simulink model "RLFactory"  (R2021a)
settings: Solver=VariableStepAuto  StartTime=0.0  StopTime=1000  RelTol=1e-3
undefined symbols (not defined in the file): BLOCKEDTIMER, GOALSA, GOALSB, GOALSRL, INITAX, INITAY, INITBX, INITBY, MAXVELOA, MAXVELOB, SAFETYDISTANCEA, SAFETYDISTANCEB, THRESHOLDA, THRESHOLDB, TSA, TSB, TSRL
libraries: rllib x1
(part 1 of 2)
settings Model: Creator=julius  LastModifiedBy=juliu
settings SolverCC: AlgebraicLoopSolver=TrustRegion
settings DebuggingCC: SFMachineParentedDataDiag=warning

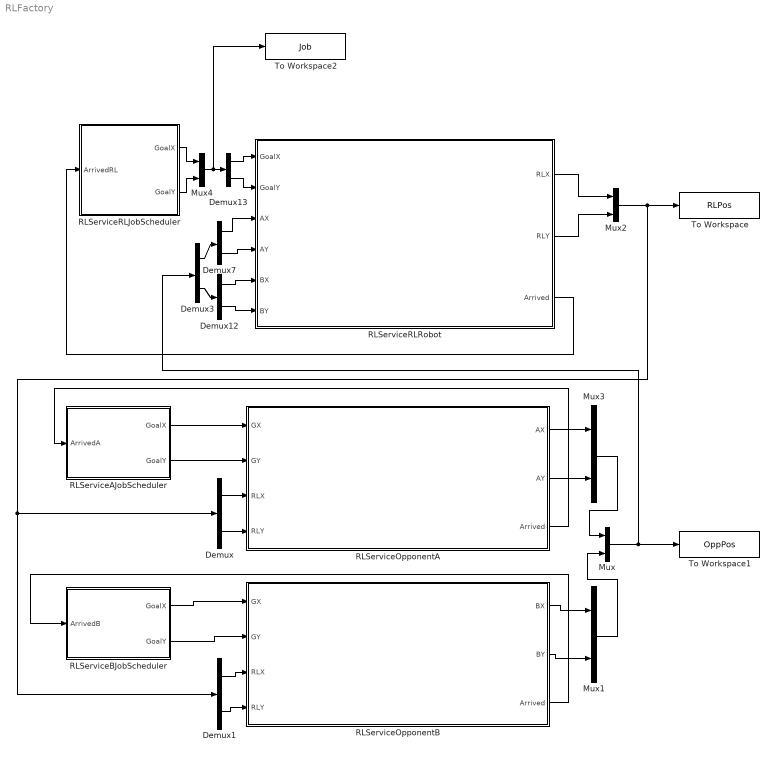
== system RLFactory ==
  Demux{,1,3,7,12..13} (6 alike) : Demux  Outputs=2
  Mux{,1..4} (5 alike) : Mux  Inputs=2
  RLServiceAJobScheduler : Subsystem
  RLServiceBJobScheduler : Subsystem
  RLServiceOpponentA : Subsystem
  RLServiceOpponentB : Subsystem
  RLServiceRLJobScheduler : Subsystem
  RLServiceRLRobot : Subsystem
  To Workspace : ToWorkspace  VariableName=RLPos  SampleTime=TSRL
  To Workspace1 : ToWorkspace  VariableName=OppPos  SampleTime=TSRL
  To Workspace2 : ToWorkspace  VariableName=Job  SampleTime=TSRL
  wires:
  RLServiceAJobScheduler/1(GoalX) -> RLServiceOpponentA/1(GX)
  RLServiceAJobScheduler/2(GoalY) -> RLServiceOpponentA/2(GY)
  RLServiceOpponentA/3(Arrived) -> RLServiceAJobScheduler/1(ArrivedA)
  Demux/1 -> RLServiceOpponentA/3(RLX)
  Demux/2 -> RLServiceOpponentA/4(RLY)
  RLServiceBJobScheduler/1(GoalX) -> RLServiceOpponentB/1(GX)
  RLServiceBJobScheduler/2(GoalY) -> RLServiceOpponentB/2(GY)
  Demux1/1 -> RLServiceOpponentB/3(RLX)
  Demux1/2 -> RLServiceOpponentB/4(RLY)
  RLServiceOpponentB/1(BX) -> Mux1/1
  RLServiceOpponentB/2(BY) -> Mux1/2
  RLServiceOpponentA/1(AX) -> Mux3/1
  RLServiceOpponentA/2(AY) -> Mux3/2
  RLServiceOpponentB/3(Arrived) -> RLServiceBJobScheduler/1(ArrivedB)
  RLServiceRLJobScheduler/2(GoalY) -> Mux4/2
  RLServiceRLJobScheduler/1(GoalX) -> Mux4/1
  Mux3/1 -> Mux/1
  Mux1/1 -> Mux/2
  Demux3/1 -> Demux7/1
  Demux3/2 -> Demux12/1
  Demux13/1 -> RLServiceRLRobot/1(GoalX)
  Demux13/2 -> RLServiceRLRobot/2(GoalY)
  Demux7/1 -> RLServiceRLRobot/3(AX)
  Demux7/2 -> RLServiceRLRobot/4(AY)
  Demux12/1 -> RLServiceRLRobot/5(BX)
  Demux12/2 -> RLServiceRLRobot/6(BY)
  RLServiceRLRobot/3(Arrived) -> RLServiceRLJobScheduler/1(ArrivedRL)
  RLServiceRLRobot/1(RLX) -> Mux2/1
  RLServiceRLRobot/2(RLY) -> Mux2/2
  Mux/1 -> To Workspace1/1, Demux3/1
  Mux2/1 -> To Workspace/1, Demux1/1, Demux/1
  Mux4/1 -> To Workspace2/1, Demux13/1

== system RLFactory/RLServiceAJobScheduler ==
  ArrivedA : Inport
  Constant1 : Constant  Value=GOALSA
  JobScheduler2 : MATLABSystem  System=JobScheduler  SimulateUsing=Interpreted execution
      mask Type: JobScheduler
      mask Display:
      | disp('JobScheduler');
      | port_label('input',1,'workstations');
      | port_label('input',2,'done');
      | port_label('output',1,'currentGoalX');
      | port_label('output',2,'currentGoalY');
  GoalX : Outport
  GoalY : Outport  Port=2
  wires:
  Constant1/1 -> JobScheduler2/1
  JobScheduler2/2 -> GoalY/1
  ArrivedA/1 -> JobScheduler2/2
  JobScheduler2/1 -> GoalX/1

== system RLFactory/RLServiceBJobScheduler ==
  ArrivedB : Inport
  Constant1 : Constant  Value=GOALSB
  JobScheduler2 : MATLABSystem  System=JobScheduler  SimulateUsing=Interpreted execution
      mask Type: JobScheduler
      mask Display:
      | disp('JobScheduler');
      | port_label('input',1,'workstations');
      | port_label('input',2,'done');
      | port_label('output',1,'currentGoalX');
      | port_label('output',2,'currentGoalY');
  GoalX : Outport
  GoalY : Outport  Port=2
  wires:
  Constant1/1 -> JobScheduler2/1
  JobScheduler2/2 -> GoalY/1
  ArrivedB/1 -> JobScheduler2/2
  JobScheduler2/1 -> GoalX/1

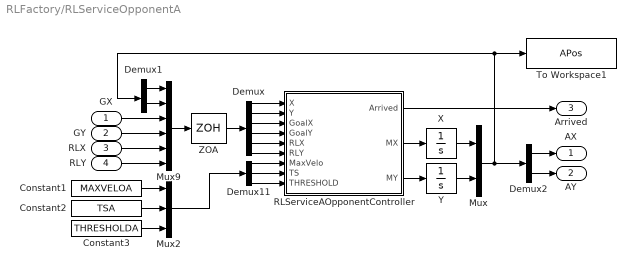
== system RLFactory/RLServiceOpponentA ==
  GX : Inport
  GY : Inport  Port=2
  RLX : Inport  Port=3
  RLY : Inport  Port=4
  Constant1 : Constant  Value=MAXVELOA
  Constant2 : Constant  Value=TSA
  Constant3 : Constant  Value=THRESHOLDA
  Demux : Demux  Outputs=6
  Demux1 : Demux  Outputs=2
  Demux11 : Demux  Outputs=3
  Demux2 : Demux  Outputs=2
  Mux : Mux  Inputs=2
  Mux2 : Mux  Inputs=3
  Mux9 : Mux  Inputs=6
  RLServiceAOpponentController : Subsystem
  To Workspace1 : ToWorkspace  VariableName=APos  SampleTime=0.25
  X : Integrator  InitialCondition=randi(INITAX)
  Y : Integrator  InitialCondition=randi(INITAY)
  ZOA : ZeroOrderHold  SampleTime=TSA
  AX : Outport
  AY : Outport  Port=2
  Arrived : Outport  Port=3
  wires:
  RLServiceAOpponentController/1(Arrived) -> Arrived/1
  Demux/4 -> RLServiceAOpponentController/4(GoalY)
  Demux/6 -> RLServiceAOpponentController/6(RLY)
  X/1 -> Mux/1
  RLY/1 -> Mux9/6
  Demux/5 -> RLServiceAOpponentController/5(RLX)
  GY/1 -> Mux9/4
  Demux/1 -> RLServiceAOpponentController/1(X)
  Y/1 -> Mux/2
  Mux/1 -> Demux1/1, To Workspace1/1, Demux2/1
  Mux9/1 -> ZOA/1
  Demux/3 -> RLServiceAOpponentController/3(GoalX)
  Demux/2 -> RLServiceAOpponentController/2(Y)
  RLX/1 -> Mux9/5
  ZOA/1 -> Demux/1
  GX/1 -> Mux9/3
  Mux2/1 -> Demux11/1
  Demux1/1 -> Mux9/1
  Demux1/2 -> Mux9/2
  Constant2/1 -> Mux2/2
  Constant1/1 -> Mux2/1
  Constant3/1 -> Mux2/3
  Demux2/1 -> AX/1
  Demux2/2 -> AY/1
  RLServiceAOpponentController/3(MY) -> Y/1
  RLServiceAOpponentController/2(MX) -> X/1
  Demux11/1 -> RLServiceAOpponentController/7(MaxVelo)
  Demux11/2 -> RLServiceAOpponentController/8(TS)
  Demux11/3 -> RLServiceAOpponentController/9(THRESHOLD)

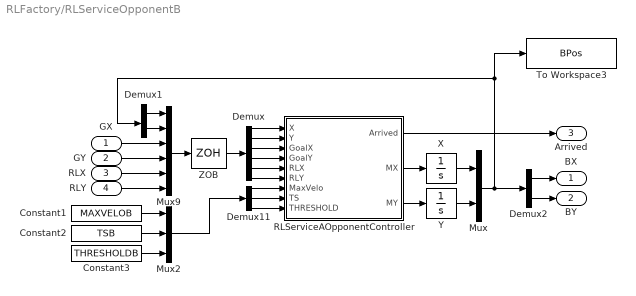
== system RLFactory/RLServiceOpponentB ==
  GX : Inport
  GY : Inport  Port=2
  RLX : Inport  Port=3
  RLY : Inport  Port=4
  Constant1 : Constant  Value=MAXVELOB
  Constant2 : Constant  Value=TSB
  Constant3 : Constant  Value=THRESHOLDB
  Demux : Demux  Outputs=6
  Demux1 : Demux  Outputs=2
  Demux11 : Demux  Outputs=3
  Demux2 : Demux  Outputs=2
  Mux : Mux  Inputs=2
  Mux2 : Mux  Inputs=3
  Mux9 : Mux  Inputs=6
  RLServiceAOpponentController : Subsystem
  To Workspace3 : ToWorkspace  VariableName=BPos  SampleTime=0.25
  X : Integrator  InitialCondition=randi(INITBX)
  Y : Integrator  InitialCondition=randi(INITBY)
  ZOB : ZeroOrderHold  SampleTime=TSB
  BX : Outport
  BY : Outport  Port=2
  Arrived : Outport  Port=3
  wires:
  RLServiceAOpponentController/3(MY) -> Y/1
  RLX/1 -> Mux9/5
  Demux11/1 -> RLServiceAOpponentController/7(MaxVelo)
  Constant2/1 -> Mux2/2
  RLServiceAOpponentController/2(MX) -> X/1
  Mux9/1 -> ZOB/1
  Constant3/1 -> Mux2/3
  Demux1/2 -> Mux9/2
  Demux/1 -> RLServiceAOpponentController/1(X)
  GY/1 -> Mux9/4
  Demux/4 -> RLServiceAOpponentController/4(GoalY)
  RLServiceAOpponentController/1(Arrived) -> Arrived/1
  X/1 -> Mux/1
  Mux/1 -> To Workspace3/1, Demux1/1, Demux2/1
  Demux/6 -> RLServiceAOpponentController/6(RLY)
  Demux/3 -> RLServiceAOpponentController/3(GoalX)
  Demux1/1 -> Mux9/1
  Demux11/2 -> RLServiceAOpponentController/8(TS)
  Demux2/1 -> BX/1
  RLY/1 -> Mux9/6
  Demux/2 -> RLServiceAOpponentController/2(Y)
  Demux11/3 -> RLServiceAOpponentController/9(THRESHOLD)
  ZOB/1 -> Demux/1
  Demux2/2 -> BY/1
  Mux2/1 -> Demux11/1
  Constant1/1 -> Mux2/1
  GX/1 -> Mux9/3
  Y/1 -> Mux/2
  Demux/5 -> RLServiceAOpponentController/5(RLX)

== system RLFactory/RLServiceRLJobScheduler ==
  ArrivedRL : Inport
  Constant : Constant  Value=GOALSRL
  JobScheduler1 : MATLABSystem  System=JobScheduler  SimulateUsing=Code generation
      mask Type: JobScheduler
      mask Display:
      | disp('JobScheduler');
      | port_label('input',1,'workstations');
      | port_label('input',2,'done');
      | port_label('output',1,'currentGoalX');
      | port_label('output',2,'currentGoalY');
  GoalX : Outport
  GoalY : Outport  Port=2
  wires:
  Constant/1 -> JobScheduler1/1
  JobScheduler1/2 -> GoalY/1
  ArrivedRL/1 -> JobScheduler1/2
  JobScheduler1/1 -> GoalX/1

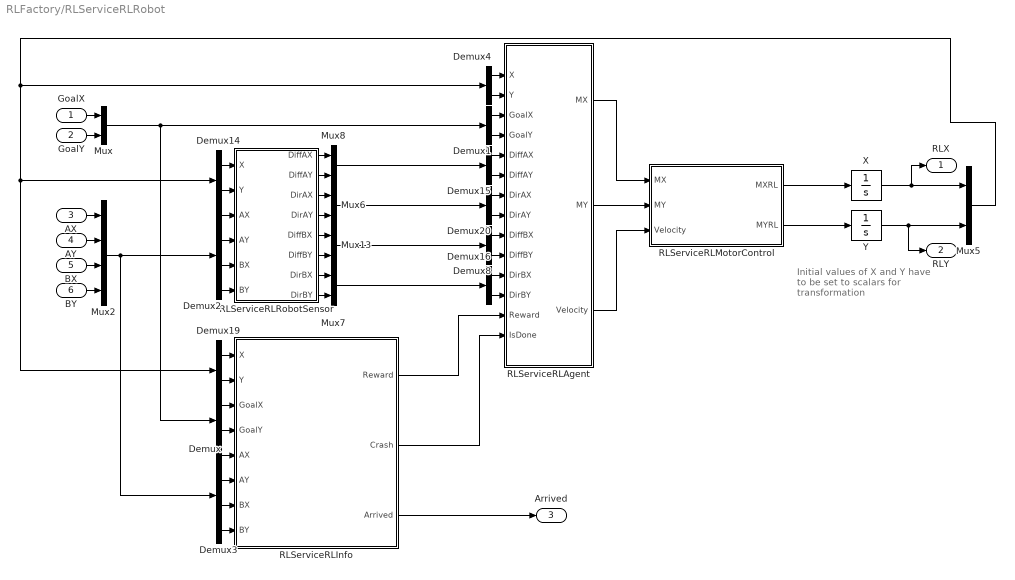
== system RLFactory/RLServiceRLRobot ==
  note: Initial values of X and Y have to be set to scalars for transformation
  GoalX : Inport
  GoalY : Inport  Port=2
  AX : Inport  Port=3
  AY : Inport  Port=4
  BX : Inport  Port=5
  BY : Inport  Port=6
  Demux{,1,4,8,14..16,19..20} (9 alike) : Demux  Outputs=2
  Demux2 : Demux
  Demux3 : Demux
  Mux{,5..8,13} (6 alike) : Mux  Inputs=2
  Mux2 : Mux
  RLServiceRLAgent : Subsystem
  RLServiceRLInfo : Subsystem
  RLServiceRLMotorControl : Subsystem
  RLServiceRLRobotSensor : Subsystem
  X : Integrator  InitialCondition=GOALSRL(1,randi(length(GOALSRL),1))
  Y : Integrator  InitialCondition=GOALSRL(2,randi(length(GOALSRL),1))
  RLX : Outport
  RLY : Outport  Port=2
  Arrived : Outport  Port=3
  wires:
  AX/1 -> Mux2/1
  X/1 -> Mux5/1, RLX/1
  Mux13/1 -> Demux8/1
  Demux2/4 -> RLServiceRLRobotSensor/6(BY)
  Demux4/1 -> RLServiceRLAgent/1(X)
  RLServiceRLRobotSensor/5(DiffBX) -> Mux13/1
  Demux4/2 -> RLServiceRLAgent/2(Y)
  Demux2/1 -> RLServiceRLRobotSensor/3(AX)
  Demux14/2 -> RLServiceRLRobotSensor/2(Y)
  Demux15/1 -> RLServiceRLAgent/5(DiffAX)
  Demux2/2 -> RLServiceRLRobotSensor/4(AY)
  RLServiceRLRobotSensor/4(DirAY) -> Mux6/2
  GoalX/1 -> Mux/1
  Demux20/2 -> RLServiceRLAgent/8(DirAY)
  RLServiceRLRobotSensor/2(DiffAY) -> Mux8/2
  RLServiceRLRobotSensor/7(DirBX) -> Mux7/1
  Mux/1 -> Demux1/1, Demux/1
  Demux2/3 -> RLServiceRLRobotSensor/5(BX)
  Demux1/2 -> RLServiceRLAgent/4(GoalY)
  Demux16/1 -> RLServiceRLAgent/11(DirBX)
  Demux15/2 -> RLServiceRLAgent/6(DiffAY)
  Demux1/1 -> RLServiceRLAgent/3(GoalX)
  Y/1 -> RLY/1, Mux5/2
  RLServiceRLRobotSensor/3(DirAX) -> Mux6/1
  RLServiceRLAgent/2(MY) -> RLServiceRLMotorControl/2(MY)
  Mux2/1 -> Demux3/1, Demux2/1
  Demux20/1 -> RLServiceRLAgent/7(DirAX)
  RLServiceRLRobotSensor/8(DirBY) -> Mux7/2
  Demux8/1 -> RLServiceRLAgent/9(DiffBX)
  BY/1 -> Mux2/4
  GoalY/1 -> Mux/2
  Mux5/1 -> Demux4/1, Demux14/1, Demux19/1
  Mux6/1 -> Demux20/1
  RLServiceRLAgent/1(MX) -> RLServiceRLMotorControl/1(MX)
  RLServiceRLRobotSensor/1(DiffAX) -> Mux8/1
  Mux7/1 -> Demux16/1
  BX/1 -> Mux2/3
  Demux16/2 -> RLServiceRLAgent/12(DirBY)
  AY/1 -> Mux2/2
  Demux8/2 -> RLServiceRLAgent/10(DiffBY)
  Mux8/1 -> Demux15/1
  Demux14/1 -> RLServiceRLRobotSensor/1(X)
  RLServiceRLRobotSensor/6(DiffBY) -> Mux13/2
  RLServiceRLAgent/3(Velocity) -> RLServiceRLMotorControl/3(Velocity)
  RLServiceRLMotorControl/1(MXRL) -> X/1
  RLServiceRLMotorControl/2(MYRL) -> Y/1
  RLServiceRLInfo/2(Crash) -> RLServiceRLAgent/14(IsDone)
  Demux19/1 -> RLServiceRLInfo/1(X)
  Demux19/2 -> RLServiceRLInfo/2(Y)
  Demux/1 -> RLServiceRLInfo/3(GoalX)
  Demux/2 -> RLServiceRLInfo/4(GoalY)
  Demux3/1 -> RLServiceRLInfo/5(AX)
  Demux3/2 -> RLServiceRLInfo/6(AY)
  Demux3/3 -> RLServiceRLInfo/7(BX)
  Demux3/4 -> RLServiceRLInfo/8(BY)
  RLServiceRLInfo/1(Reward) -> RLServiceRLAgent/13(Reward)
  RLServiceRLInfo/3(Arrived) -> Arrived/1

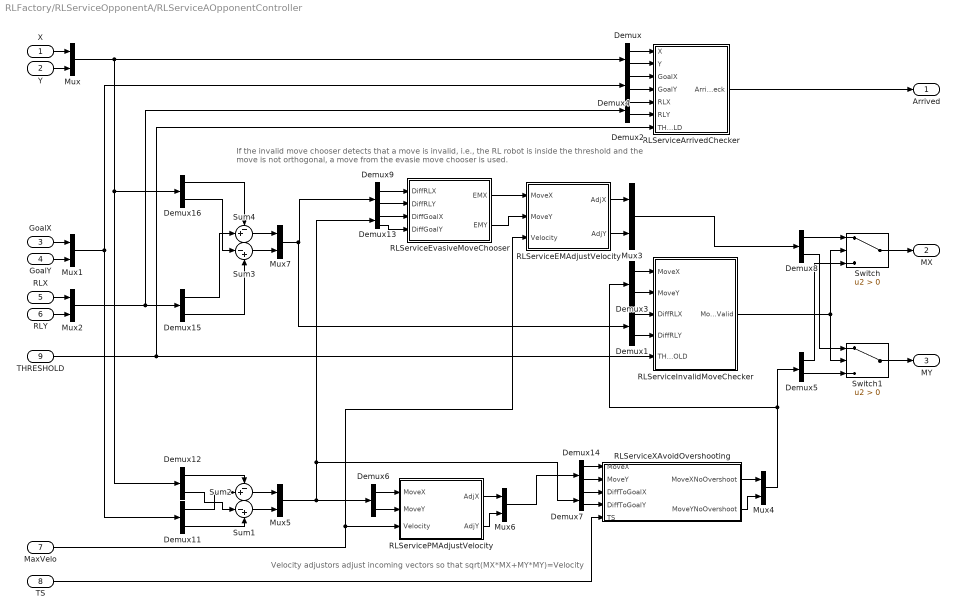
== system RLFactory/RLServiceOpponentA/RLServiceAOpponentController ==
  note: If the invalid move chooser detects that a move is invalid, i.e.,
      | the RL robot is inside the threshold and the move is not orthogonal, a move from the evasie move chooser is used.
  note: Velocity adjustors adjust incoming vectors so that sqrt(MX*MX+MY*MY)=Velocity
  X : Inport
  Y : Inport  Port=2
  GoalX : Inport  Port=3
  GoalY : Inport  Port=4
  RLX : Inport  Port=5
  RLY : Inport  Port=6
  MaxVelo : Inport  Port=7
  TS : Inport  Port=8
  THRESHOLD : Inport  Port=9
  Demux{,1..9,11..16} (16 alike) : Demux  Outputs=2
  Mux{,1..7} (8 alike) : Mux  Inputs=2
  RLServiceArrivedChecker : Subsystem
  RLServiceEMAdjustVelocity : Subsystem
  RLServiceEvasiveMoveChooser : Subsystem
  RLServiceInvalidMoveChecker : Subsystem
  RLServicePMAdjustVelocity : Subsystem
  RLServiceXAvoidOvershooting : Subsystem
  Sum1 : Sum  Inputs=|-+
  Sum2 : Sum  Inputs=-+|
  Sum3 : Sum  Inputs=|-+
  Sum4 : Sum  Inputs=-+|
  Switch : Switch  Criteria=u2 > Threshold
  Switch1 : Switch  Criteria=u2 > Threshold
  Arrived : Outport
  MX : Outport  Port=2
  MY : Outport  Port=3
  wires:
  GoalX/1 -> Mux1/1
  GoalY/1 -> Mux1/2
  RLServiceArrivedChecker/1(ArrivedCheck) -> Arrived/1
  Demux/1 -> RLServiceArrivedChecker/1(X)
  Demux/2 -> RLServiceArrivedChecker/2(Y)
  Demux4/1 -> RLServiceArrivedChecker/3(GoalX)
  Demux4/2 -> RLServiceArrivedChecker/4(GoalY)
  X/1 -> Mux/1
  Y/1 -> Mux/2
  RLX/1 -> Mux2/1
  RLY/1 -> Mux2/2
  Demux3/1 -> RLServiceInvalidMoveChecker/1(MoveX)
  Demux8/1 -> Switch/1
  Demux5/2 -> Switch1/3
  Demux8/2 -> Switch1/1
  THRESHOLD/1 -> RLServiceArrivedChecker/7(THRESHOLD), RLServiceInvalidMoveChecker/5(THRESHOLD)
  Demux3/2 -> RLServiceInvalidMoveChecker/2(MoveY)
  Demux5/1 -> Switch/3
  RLServiceInvalidMoveChecker/1(MoveInValid) -> Switch/2, Switch1/2
  Switch/1 -> MX/1
  Switch1/1 -> MY/1
  Mux5/1 -> Demux6/1, Demux7/1, Demux13/1
  Demux6/2 -> RLServicePMAdjustVelocity/2(MoveY)
  Mux1/1 -> Demux4/1, Demux11/1
  TS/1 -> RLServiceXAvoidOvershooting/5(TS)
  MaxVelo/1 -> RLServiceEMAdjustVelocity/3(Velocity), RLServicePMAdjustVelocity/3(Velocity)
  RLServicePMAdjustVelocity/1(AdjX) -> Mux6/1
  RLServicePMAdjustVelocity/2(AdjY) -> Mux6/2
  RLServiceEvasiveMoveChooser/1(EMX) -> RLServiceEMAdjustVelocity/1(MoveX)
  RLServiceEvasiveMoveChooser/2(EMY) -> RLServiceEMAdjustVelocity/2(MoveY)
  RLServiceEMAdjustVelocity/1(AdjX) -> Mux3/1
  RLServiceEMAdjustVelocity/2(AdjY) -> Mux3/2
  Mux3/1 -> Demux8/1
  RLServiceXAvoidOvershooting/1(MoveXNoOvershoot) -> Mux4/1
  RLServiceXAvoidOvershooting/2(MoveYNoOvershoot) -> Mux4/2
  Mux4/1 -> Demux5/1, Demux3/1
  Sum2/1 -> Mux5/1
  Sum1/1 -> Mux5/2
  Demux6/1 -> RLServicePMAdjustVelocity/1(MoveX)
  Demux7/1 -> RLServiceXAvoidOvershooting/3(DiffToGoalX)
  Demux7/2 -> RLServiceXAvoidOvershooting/4(DiffToGoalY)
  Demux13/1 -> RLServiceEvasiveMoveChooser/3(DiffGoalX)
  Demux13/2 -> RLServiceEvasiveMoveChooser/4(DiffGoalY)
  Demux11/1 -> Sum2/2
  Demux12/2 -> Sum1/1
  Demux11/2 -> Sum1/2
  Demux12/1 -> Sum2/1
  Demux14/1 -> RLServiceXAvoidOvershooting/1(MoveX)
  Demux14/2 -> RLServiceXAvoidOvershooting/2(MoveY)
  Mux6/1 -> Demux14/1
  Sum3/1 -> Mux7/2
  Demux16/1 -> Sum4/1
  Sum4/1 -> Mux7/1
  Mux/1 -> Demux12/1, Demux16/1, Demux/1
  Mux2/1 -> Demux2/1, Demux15/1
  Demux15/2 -> Sum3/2
  Demux15/1 -> Sum4/2
  Demux16/2 -> Sum3/1
  Demux9/1 -> RLServiceEvasiveMoveChooser/1(DiffRLX)
  Demux9/2 -> RLServiceEvasiveMoveChooser/2(DiffRLY)
  Mux7/1 -> Demux1/1, Demux9/1
  Demux1/1 -> RLServiceInvalidMoveChecker/3(DiffRLX)
  Demux1/2 -> RLServiceInvalidMoveChecker/4(DiffRLY)
  Demux2/2 -> RLServiceArrivedChecker/6(RLY)
  Demux2/1 -> RLServiceArrivedChecker/5(RLX)

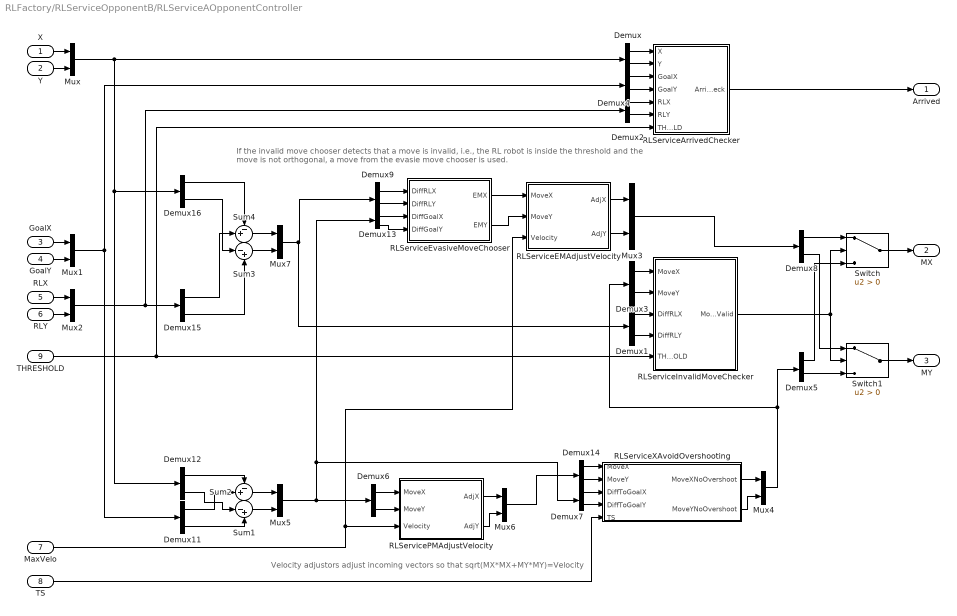
== system RLFactory/RLServiceOpponentB/RLServiceAOpponentController ==
  note: If the invalid move chooser detects that a move is invalid, i.e.,
      | the RL robot is inside the threshold and the move is not orthogonal, a move from the evasie move chooser is used.
  note: Velocity adjustors adjust incoming vectors so that sqrt(MX*MX+MY*MY)=Velocity
  X : Inport
  Y : Inport  Port=2
  GoalX : Inport  Port=3
  GoalY : Inport  Port=4
  RLX : Inport  Port=5
  RLY : Inport  Port=6
  MaxVelo : Inport  Port=7
  TS : Inport  Port=8
  THRESHOLD : Inport  Port=9
  Demux{,1..9,11..16} (16 alike) : Demux  Outputs=2
  Mux{,1..7} (8 alike) : Mux  Inputs=2
  RLServiceArrivedChecker : Subsystem
  RLServiceEMAdjustVelocity : Subsystem
  RLServiceEvasiveMoveChooser : Subsystem
  RLServiceInvalidMoveChecker : Subsystem
  RLServicePMAdjustVelocity : Subsystem
  RLServiceXAvoidOvershooting : Subsystem
  Sum1 : Sum  Inputs=|-+
  Sum2 : Sum  Inputs=-+|
  Sum3 : Sum  Inputs=|-+
  Sum4 : Sum  Inputs=-+|
  Switch : Switch  Criteria=u2 > Threshold
  Switch1 : Switch  Criteria=u2 > Threshold
  Arrived : Outport
  MX : Outport  Port=2
  MY : Outport  Port=3
  wires:
  GoalX/1 -> Mux1/1
  GoalY/1 -> Mux1/2
  RLServiceArrivedChecker/1(ArrivedCheck) -> Arrived/1
  Demux/1 -> RLServiceArrivedChecker/1(X)
  Demux/2 -> RLServiceArrivedChecker/2(Y)
  Demux4/1 -> RLServiceArrivedChecker/3(GoalX)
  Demux4/2 -> RLServiceArrivedChecker/4(GoalY)
  X/1 -> Mux/1
  Y/1 -> Mux/2
  RLX/1 -> Mux2/1
  RLY/1 -> Mux2/2
  Demux3/1 -> RLServiceInvalidMoveChecker/1(MoveX)
  Demux8/1 -> Switch/1
  Demux5/2 -> Switch1/3
  Demux8/2 -> Switch1/1
  THRESHOLD/1 -> RLServiceArrivedChecker/7(THRESHOLD), RLServiceInvalidMoveChecker/5(THRESHOLD)
  Demux3/2 -> RLServiceInvalidMoveChecker/2(MoveY)
  Demux5/1 -> Switch/3
  RLServiceInvalidMoveChecker/1(MoveInValid) -> Switch/2, Switch1/2
  Switch/1 -> MX/1
  Switch1/1 -> MY/1
  Mux5/1 -> Demux6/1, Demux7/1, Demux13/1
  Demux6/2 -> RLServicePMAdjustVelocity/2(MoveY)
  Mux1/1 -> Demux4/1, Demux11/1
  TS/1 -> RLServiceXAvoidOvershooting/5(TS)
  MaxVelo/1 -> RLServiceEMAdjustVelocity/3(Velocity), RLServicePMAdjustVelocity/3(Velocity)
  RLServicePMAdjustVelocity/1(AdjX) -> Mux6/1
  RLServicePMAdjustVelocity/2(AdjY) -> Mux6/2
  RLServiceEvasiveMoveChooser/1(EMX) -> RLServiceEMAdjustVelocity/1(MoveX)
  RLServiceEvasiveMoveChooser/2(EMY) -> RLServiceEMAdjustVelocity/2(MoveY)
  RLServiceEMAdjustVelocity/1(AdjX) -> Mux3/1
  RLServiceEMAdjustVelocity/2(AdjY) -> Mux3/2
  Mux3/1 -> Demux8/1
  RLServiceXAvoidOvershooting/1(MoveXNoOvershoot) -> Mux4/1
  RLServiceXAvoidOvershooting/2(MoveYNoOvershoot) -> Mux4/2
  Mux4/1 -> Demux5/1, Demux3/1
  Sum2/1 -> Mux5/1
  Sum1/1 -> Mux5/2
  Demux6/1 -> RLServicePMAdjustVelocity/1(MoveX)
  Demux7/1 -> RLServiceXAvoidOvershooting/3(DiffToGoalX)
  Demux7/2 -> RLServiceXAvoidOvershooting/4(DiffToGoalY)
  Demux13/1 -> RLServiceEvasiveMoveChooser/3(DiffGoalX)
  Demux13/2 -> RLServiceEvasiveMoveChooser/4(DiffGoalY)
  Demux11/1 -> Sum2/2
  Demux12/2 -> Sum1/1
  Demux11/2 -> Sum1/2
  Demux12/1 -> Sum2/1
  Demux14/1 -> RLServiceXAvoidOvershooting/1(MoveX)
  Demux14/2 -> RLServiceXAvoidOvershooting/2(MoveY)
  Mux6/1 -> Demux14/1
  Sum3/1 -> Mux7/2
  Demux16/1 -> Sum4/1
  Sum4/1 -> Mux7/1
  Mux/1 -> Demux12/1, Demux16/1, Demux/1
  Mux2/1 -> Demux2/1, Demux15/1
  Demux15/2 -> Sum3/2
  Demux15/1 -> Sum4/2
  Demux16/2 -> Sum3/1
  Demux9/1 -> RLServiceEvasiveMoveChooser/1(DiffRLX)
  Demux9/2 -> RLServiceEvasiveMoveChooser/2(DiffRLY)
  Mux7/1 -> Demux1/1, Demux9/1
  Demux1/1 -> RLServiceInvalidMoveChecker/3(DiffRLX)
  Demux1/2 -> RLServiceInvalidMoveChecker/4(DiffRLY)
  Demux2/2 -> RLServiceArrivedChecker/6(RLY)
  Demux2/1 -> RLServiceArrivedChecker/5(RLX)

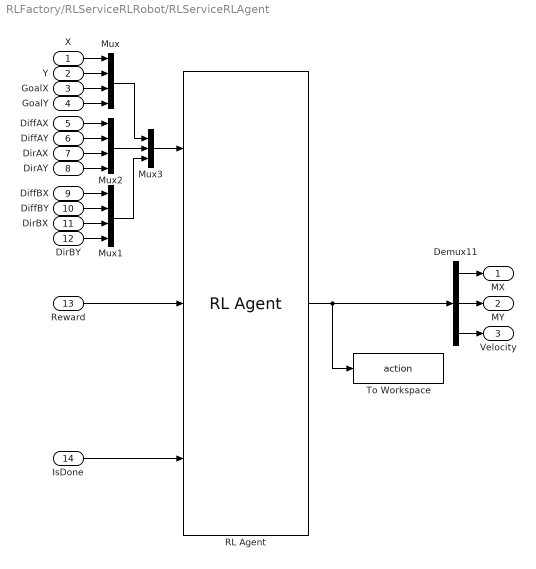
== system RLFactory/RLServiceRLRobot/RLServiceRLAgent ==
  X : Inport
  Y : Inport  Port=2
  GoalX : Inport  Port=3
  GoalY : Inport  Port=4
  DiffAX : Inport  Port=5
  DiffAY : Inport  Port=6
  DirAX : Inport  Port=7
  DirAY : Inport  Port=8
  DiffBX : Inport  Port=9
  DiffBY : Inport  Port=10
  DirBX : Inport  Port=11
  DirBY : Inport  Port=12
  Reward : Inport  Port=13
  IsDone : Inport  Port=14
  Demux11 : Demux  Outputs=3
  Mux : Mux
  Mux1 : Mux
  Mux2 : Mux
  Mux3 : Mux  Inputs=3
  RL Agent : rllib/RL Agent  Agent=qAgent  ProvideReward=on  ProvideIsDone=on  ProvideCumRwd=off  TreatAsDirectFeedthrough=on  CollectLoggedSignals=on  CollectModelStates=on
  To Workspace : ToWorkspace  VariableName=action  SampleTime=-1
  MX : Outport
  MY : Outport  Port=2
  Velocity : Outport  Port=3
  wires:
  IsDone/1 -> RL Agent/3
  Demux11/1 -> MX/1
  Reward/1 -> RL Agent/2
  DirAX/1 -> Mux2/3
  GoalY/1 -> Mux/4
  DiffAX/1 -> Mux2/1
  X/1 -> Mux/1
  GoalX/1 -> Mux/3
  DirAY/1 -> Mux2/4
  DiffAY/1 -> Mux2/2
  Y/1 -> Mux/2
  DiffBX/1 -> Mux1/1
  DiffBY/1 -> Mux1/2
  DirBX/1 -> Mux1/3
  DirBY/1 -> Mux1/4
  Mux2/1 -> Mux3/2
  Mux3/1 -> RL Agent/1
  Mux/1 -> Mux3/1
  Mux1/1 -> Mux3/3
  RL Agent/1 -> To Workspace/1, Demux11/1
  Demux11/2 -> MY/1
  Demux11/3 -> Velocity/1

== system RLFactory/RLServiceRLRobot/RLServiceRLInfo ==
  X : Inport
  Y : Inport  Port=2
  GoalX : Inport  Port=3
  GoalY : Inport  Port=4
  AX : Inport  Port=5
  AY : Inport  Port=6
  BX : Inport  Port=7
  BY : Inport  Port=8
  RLServiceCrashDetector : Subsystem
  RLServiceGoalTracker : Subsystem
  RLServiceReward : Subsystem
  To Workspace1 : ToWorkspace  VariableName=Crash  SampleTime=-1
      settings: MaxDataPoints=1
  Reward : Outport
  Crash : Outport  Port=2
  Arrived : Outport  Port=3
  wires:
  BY/1 -> RLServiceCrashDetector/6(BY)
  GoalY/1 -> RLServiceGoalTracker/4(GoalY)
  AX/1 -> RLServiceCrashDetector/3(AX)
  RLServiceGoalTracker/2(Arrived) -> Arrived/1, RLServiceReward/2(Arrived)
  Y/1 -> RLServiceGoalTracker/2(Y), RLServiceCrashDetector/2(Y)
  GoalX/1 -> RLServiceGoalTracker/3(GoalX)
  BX/1 -> RLServiceCrashDetector/5(BX)
  RLServiceReward/1(Reward) -> Reward/1
  AY/1 -> RLServiceCrashDetector/4(AY)
  X/1 -> RLServiceGoalTracker/1(X), RLServiceCrashDetector/1(X)
  RLServiceGoalTracker/1(Dist) -> RLServiceReward/1(DistGoal)
  RLServiceCrashDetector/2(Crash) -> To Workspace1/1, RLServiceReward/3(Crash), Crash/1
  RLServiceCrashDetector/1(BelowThreshold) -> RLServiceReward/4(BelowThreshold)

== system RLFactory/RLServiceRLRobot/RLServiceRLMotorControl ==
  MX : Inport
  MY : Inport  Port=2
  Velocity : Inport  Port=3
  RLServiceRLAdjustVelocity : Subsystem
  MXRL : Outport
  MYRL : Outport  Port=2
  wires:
  RLServiceRLAdjustVelocity/1(AdjMX) -> MXRL/1
  RLServiceRLAdjustVelocity/2(AdjMY) -> MYRL/1
  MX/1 -> RLServiceRLAdjustVelocity/1(MoveX)
  MY/1 -> RLServiceRLAdjustVelocity/2(MoveY)
  Velocity/1 -> RLServiceRLAdjustVelocity/3(Velocity)

== system RLFactory/RLServiceRLRobot/RLServiceRLRobotSensor ==
  X : Inport
  Y : Inport  Port=2
  AX : Inport  Port=3
  AY : Inport  Port=4
  BX : Inport  Port=5
  BY : Inport  Port=6
  RLServiceARobotSensorSubsystem : Subsystem
  RLServiceBRobotSensorSubsystem : Subsystem
  DiffAX : Outport
  DiffAY : Outport  Port=2
  DirAX : Outport  Port=3
  DirAY : Outport  Port=4
  DiffBX : Outport  Port=5
  DiffBY : Outport  Port=6
  DirBX : Outport  Port=7
  DirBY : Outport  Port=8
  wires:
  RLServiceBRobotSensorSubsystem/3(DirOppX) -> DirBX/1
  BY/1 -> RLServiceBRobotSensorSubsystem/4(OppY)
  BX/1 -> RLServiceBRobotSensorSubsystem/3(OppX)
  RLServiceARobotSensorSubsystem/4(DirOppY) -> DirAY/1
  X/1 -> RLServiceBRobotSensorSubsystem/1(X), RLServiceARobotSensorSubsystem/1(X)
  RLServiceBRobotSensorSubsystem/4(DirOppY) -> DirBY/1
  Y/1 -> RLServiceBRobotSensorSubsystem/2(Y), RLServiceARobotSensorSubsystem/2(Y)
  RLServiceBRobotSensorSubsystem/2(DiffOppY) -> DiffBY/1
  RLServiceARobotSensorSubsystem/3(DirOppX) -> DirAX/1
  RLServiceBRobotSensorSubsystem/1(DiffOppX) -> DiffBX/1
  AX/1 -> RLServiceARobotSensorSubsystem/3(OppX)
  AY/1 -> RLServiceARobotSensorSubsystem/4(OppY)
  RLServiceARobotSensorSubsystem/1(DiffOppX) -> DiffAX/1
  RLServiceARobotSensorSubsystem/2(DiffOppY) -> DiffAY/1

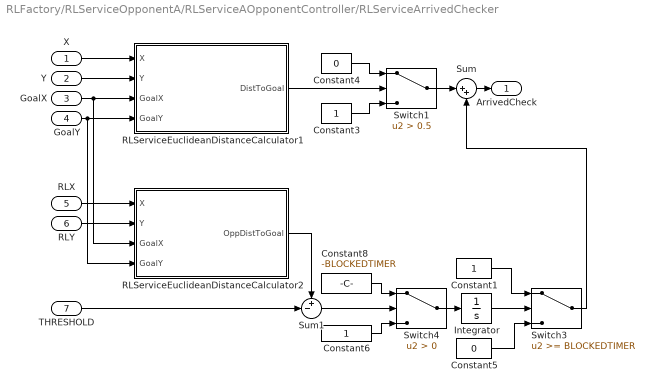
== system RLFactory/RLServiceOpponentA/RLServiceAOpponentController/RLServiceArrivedChecker ==
  X : Inport
  Y : Inport  Port=2
  GoalX : Inport  Port=3
  GoalY : Inport  Port=4
  RLX : Inport  Port=5
  RLY : Inport  Port=6
  THRESHOLD : Inport  Port=7
  Constant1 : Constant
  Constant3 : Constant
  Constant4 : Constant  Value=0
  Constant5 : Constant  Value=0
  Constant6 : Constant
  Constant8 : Constant  Value=-BLOCKEDTIMER
  Integrator : Integrator  LimitOutput=on  UpperSaturationLimit=BLOCKEDTIMER  LowerSaturationLimit=0
  RLServiceEuclideanDistanceCalculator1 : Subsystem
  RLServiceEuclideanDistanceCalculator2 : Subsystem
  Sum : Sum  Inputs=|++
  Sum1 : Sum  Inputs=+-|
  Switch1 : Switch  Criteria=u2 > Threshold  Threshold=0.5
  Switch3 : Switch  Threshold=BLOCKEDTIMER
  Switch4 : Switch  Criteria=u2 > Threshold
  ArrivedCheck : Outport
  wires:
  RLServiceEuclideanDistanceCalculator1/1(DistToGoal) -> Switch1/2
  X/1 -> RLServiceEuclideanDistanceCalculator1/1(X)
  Switch1/1 -> Sum/1
  Constant3/1 -> Switch1/3
  Y/1 -> RLServiceEuclideanDistanceCalculator1/2(Y)
  Constant4/1 -> Switch1/1
  Sum/1 -> ArrivedCheck/1
  Switch3/1 -> Sum/2
  Integrator/1 -> Switch3/2
  Constant5/1 -> Switch3/3
  RLX/1 -> RLServiceEuclideanDistanceCalculator2/1(X)
  RLY/1 -> RLServiceEuclideanDistanceCalculator2/2(Y)
  GoalX/1 -> RLServiceEuclideanDistanceCalculator2/3(GoalX), RLServiceEuclideanDistanceCalculator1/3(GoalX)
  GoalY/1 -> RLServiceEuclideanDistanceCalculator2/4(GoalY), RLServiceEuclideanDistanceCalculator1/4(GoalY)
  RLServiceEuclideanDistanceCalculator2/1(OppDistToGoal) -> Sum1/1
  Constant8/1 -> Switch4/1
  Constant6/1 -> Switch4/3
  THRESHOLD/1 -> Sum1/2
  Sum1/1 -> Switch4/2
  Switch4/1 -> Integrator/1
  Constant1/1 -> Switch3/1

== system RLFactory/RLServiceOpponentA/RLServiceAOpponentController/RLServiceEMAdjustVelocity ==
  MoveX : Inport
  MoveY : Inport  Port=2
  Velocity : Inport  Port=3
  Constant : Constant
  Demux1 : Demux  Outputs=2
  Divide : Product  Inputs=*/
  Divide1 : Product  Inputs=*/
  Mux : Mux  Inputs=2
  Product : Product
  Product3 : Product
  Sqrt1 : Sqrt  SaturateOnIntegerOverflow=on
  Square : Math  Operator=square  SaturateOnIntegerOverflow=on
  Square1 : Math  Operator=square  SaturateOnIntegerOverflow=on
  Sum : Sum  Inputs=+|+
  Switch : Switch  Criteria=u2 > Threshold
  AdjX : Outport
  AdjY : Outport  Port=2
  wires:
  Product/1 -> AdjX/1
  MoveY/1 -> Square1/1, Mux/2
  Mux/1 -> Demux1/1
  Divide1/1 -> Product3/1
  Constant/1 -> Switch/3
  Square1/1 -> Sum/2
  Switch/1 -> Divide1/2, Divide/2
  Velocity/1 -> Product/2, Product3/2
  Sum/1 -> Sqrt1/1
  Square/1 -> Sum/1
  Sqrt1/1 -> Switch/2, Switch/1
  Product3/1 -> AdjY/1
  Demux1/2 -> Divide1/1
  MoveX/1 -> Square/1, Mux/1
  Demux1/1 -> Divide/1
  Divide/1 -> Product/1

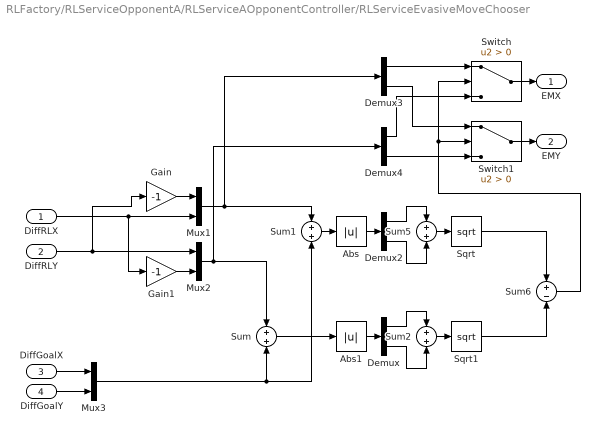
== system RLFactory/RLServiceOpponentA/RLServiceAOpponentController/RLServiceEvasiveMoveChooser ==
  DiffRLX : Inport
  DiffRLY : Inport  Port=2
  DiffGoalX : Inport  Port=3
  DiffGoalY : Inport  Port=4
  Abs : Abs
  Abs1 : Abs
  Demux{,2..4} (4 alike) : Demux  Outputs=2
  Gain : Gain  Gain=-1
  Gain1 : Gain  Gain=-1
  Mux1 : Mux  Inputs=2
  Mux2 : Mux  Inputs=2
  Mux3 : Mux  Inputs=2
  Sqrt : Sqrt  SaturateOnIntegerOverflow=on
  Sqrt1 : Sqrt  SaturateOnIntegerOverflow=on
  Sum{,1..2,5} (4 alike) : Sum  Inputs=+|+
  Sum6 : Sum  Inputs=+|-
  Switch : Switch  Criteria=u2 > Threshold
  Switch1 : Switch  Criteria=u2 > Threshold
  EMX : Outport
  EMY : Outport  Port=2
  wires:
  Gain/1 -> Mux1/1
  DiffRLX/1 -> Gain1/1, Mux1/2
  Gain1/1 -> Mux2/2
  DiffGoalX/1 -> Mux3/1
  DiffGoalY/1 -> Mux3/2
  Mux3/1 -> Sum/2, Sum1/2
  Mux2/1 -> Sum/1, Demux4/1
  Mux1/1 -> Demux3/1, Sum1/1
  Sum1/1 -> Abs/1
  Sum/1 -> Abs1/1
  Abs1/1 -> Demux/1
  Demux/1 -> Sum2/1
  Demux/2 -> Sum2/2
  Demux2/2 -> Sum5/2
  Demux2/1 -> Sum5/1
  Abs/1 -> Demux2/1
  Sum5/1 -> Sqrt/1
  Sum2/1 -> Sqrt1/1
  Sqrt/1 -> Sum6/1
  Sqrt1/1 -> Sum6/2
  Sum6/1 -> Switch/2, Switch1/2
  Demux3/1 -> Switch/1
  Demux3/2 -> Switch1/1
  Demux4/1 -> Switch/3
  Demux4/2 -> Switch1/3
  Switch/1 -> EMX/1
  Switch1/1 -> EMY/1
  DiffRLY/1 -> Mux2/1, Gain/1

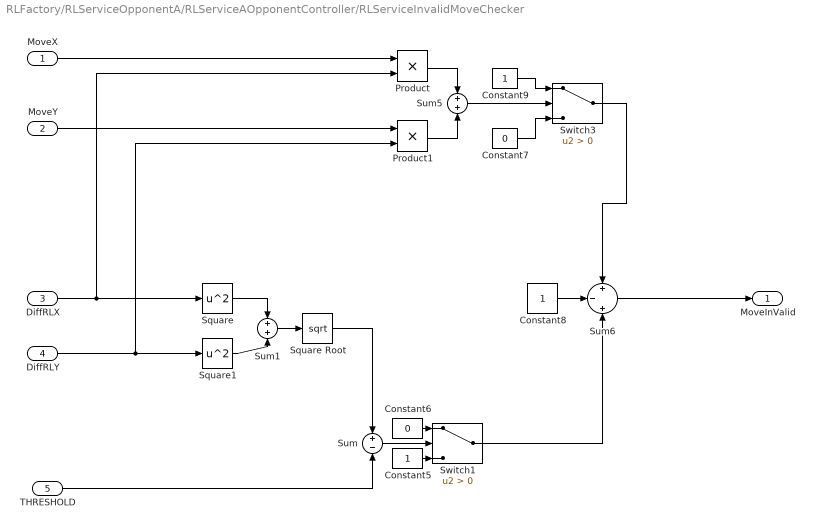
== system RLFactory/RLServiceOpponentA/RLServiceAOpponentController/RLServiceInvalidMoveChecker ==
  MoveX : Inport
  MoveY : Inport  Port=2
  DiffRLX : Inport  Port=3
  DiffRLY : Inport  Port=4
  THRESHOLD : Inport  Port=5
  Constant5 : Constant
  Constant6 : Constant  Value=0
  Constant7 : Constant  Value=0
  Constant8 : Constant
  Constant9 : Constant
  Product : Product
  Product1 : Product
  Square : Math  Operator=square  SaturateOnIntegerOverflow=on
  Square Root : Sqrt  SaturateOnIntegerOverflow=on
  Square1 : Math  Operator=square  SaturateOnIntegerOverflow=on
  Sum : Sum  Inputs=+|-
  Sum1 : Sum
  Sum5 : Sum  Inputs=+|+
  Sum6 : Sum  Inputs=+|-|+
  Switch1 : Switch  Criteria=u2 > Threshold
  Switch3 : Switch  Criteria=u2 > Threshold
  MoveInValid : Outport
  wires:
  Product1/1 -> Sum5/2
  Sum5/1 -> Switch3/2
  Product/1 -> Sum5/1
  Sum6/1 -> MoveInValid/1
  Switch3/1 -> Sum6/1
  Constant9/1 -> Switch3/1
  MoveY/1 -> Product1/1
  MoveX/1 -> Product/1
  Constant8/1 -> Sum6/2
  Constant7/1 -> Switch3/3
  THRESHOLD/1 -> Sum/2
  Sum/1 -> Switch1/2
  Constant5/1 -> Switch1/3
  Constant6/1 -> Switch1/1
  Switch1/1 -> Sum6/3
  DiffRLY/1 -> Square1/1, Product1/2
  DiffRLX/1 -> Product/2, Square/1
  Square1/1 -> Sum1/2
  Sum1/1 -> Square Root/1
  Square/1 -> Sum1/1
  Square Root/1 -> Sum/1

== system RLFactory/RLServiceOpponentA/RLServiceAOpponentController/RLServicePMAdjustVelocity ==
  MoveX : Inport
  MoveY : Inport  Port=2
  Velocity : Inport  Port=3
  Constant : Constant
  Demux1 : Demux  Outputs=2
  Divide : Product  Inputs=*/
  Divide1 : Product  Inputs=*/
  Mux : Mux  Inputs=2
  Product : Product
  Product3 : Product
  Sqrt1 : Sqrt  SaturateOnIntegerOverflow=on
  Square : Math  Operator=square  SaturateOnIntegerOverflow=on
  Square1 : Math  Operator=square  SaturateOnIntegerOverflow=on
  Sum : Sum  Inputs=+|+
  Switch : Switch  Criteria=u2 > Threshold
  AdjX : Outport
  AdjY : Outport  Port=2
  wires:
  Velocity/1 -> Product/2, Product3/2
  MoveX/1 -> Square/1, Mux/1
  MoveY/1 -> Square1/1, Mux/2
  Divide1/1 -> Product3/1
  Divide/1 -> Product/1
  Switch/1 -> Divide1/2, Divide/2
  Constant/1 -> Switch/3
  Mux/1 -> Demux1/1
  Demux1/2 -> Divide1/1
  Square1/1 -> Sum/2
  Sum/1 -> Sqrt1/1
  Demux1/1 -> Divide/1
  Product/1 -> AdjX/1
  Sqrt1/1 -> Switch/2, Switch/1
  Product3/1 -> AdjY/1
  Square/1 -> Sum/1

== system RLFactory/RLServiceOpponentA/RLServiceAOpponentController/RLServiceXAvoidOvershooting ==
  MoveX : Inport
  MoveY : Inport  Port=2
  DiffToGoalX : Inport  Port=3
  DiffToGoalY : Inport  Port=4
  TS : Inport  Port=5
  Abs{1..4} (4 alike) : Abs
  Divide : Product  Inputs=*/
  Divide1 : Product  Inputs=*/
  Product : Product
  Product1 : Product
  Sum1 : Sum  Inputs=-|+
  Sum2 : Sum  Inputs=-|+
  Switch : Switch  Criteria=u2 > Threshold
  Switch1 : Switch  Criteria=u2 > Threshold
  MoveXNoOvershoot : Outport
  MoveYNoOvershoot : Outport  Port=2
  wires:
  Abs1/1 -> Sum1/2
  Switch/1 -> MoveXNoOvershoot/1
  Product/1 -> Abs2/1
  Abs2/1 -> Sum1/1
  DiffToGoalX/1 -> Divide/1, Abs1/1
  Sum1/1 -> Switch/2
  MoveX/1 -> Product/1, Switch/1
  Divide/1 -> Switch/3
  MoveY/1 -> Product1/1, Switch1/1
  Sum2/1 -> Switch1/2
  Abs4/1 -> Sum2/1
  Product1/1 -> Abs4/1
  Divide1/1 -> Switch1/3
  TS/1 -> Divide1/2, Product1/2, Divide/2, Product/2
  Abs3/1 -> Sum2/2
  Switch1/1 -> MoveYNoOvershoot/1
  DiffToGoalY/1 -> Divide1/1, Abs3/1

== system RLFactory/RLServiceOpponentB/RLServiceAOpponentController/RLServiceArrivedChecker ==
  X : Inport
  Y : Inport  Port=2
  GoalX : Inport  Port=3
  GoalY : Inport  Port=4
  RLX : Inport  Port=5
  RLY : Inport  Port=6
  THRESHOLD : Inport  Port=7
  Constant1 : Constant
  Constant3 : Constant
  Constant4 : Constant  Value=0
  Constant5 : Constant  Value=0
  Constant6 : Constant
  Constant8 : Constant  Value=-BLOCKEDTIMER
  Integrator : Integrator  LimitOutput=on  UpperSaturationLimit=BLOCKEDTIMER  LowerSaturationLimit=0
  RLServiceEuclideanDistanceCalculator1 : Subsystem
  RLServiceEuclideanDistanceCalculator2 : Subsystem
  Sum : Sum  Inputs=|++
  Sum1 : Sum  Inputs=+-|
  Switch1 : Switch  Criteria=u2 > Threshold  Threshold=0.5
  Switch3 : Switch  Threshold=BLOCKEDTIMER
  Switch4 : Switch  Criteria=u2 > Threshold
  ArrivedCheck : Outport
  wires:
  RLServiceEuclideanDistanceCalculator1/1(DistToGoal) -> Switch1/2
  X/1 -> RLServiceEuclideanDistanceCalculator1/1(X)
  Switch1/1 -> Sum/1
  Constant3/1 -> Switch1/3
  Y/1 -> RLServiceEuclideanDistanceCalculator1/2(Y)
  Constant4/1 -> Switch1/1
  Sum/1 -> ArrivedCheck/1
  Switch3/1 -> Sum/2
  Integrator/1 -> Switch3/2
  Constant5/1 -> Switch3/3
  RLX/1 -> RLServiceEuclideanDistanceCalculator2/1(X)
  RLY/1 -> RLServiceEuclideanDistanceCalculator2/2(Y)
  GoalX/1 -> RLServiceEuclideanDistanceCalculator2/3(GoalX), RLServiceEuclideanDistanceCalculator1/3(GoalX)
  GoalY/1 -> RLServiceEuclideanDistanceCalculator2/4(GoalY), RLServiceEuclideanDistanceCalculator1/4(GoalY)
  RLServiceEuclideanDistanceCalculator2/1(OppDistToGoal) -> Sum1/1
  Constant8/1 -> Switch4/1
  Constant6/1 -> Switch4/3
  THRESHOLD/1 -> Sum1/2
  Sum1/1 -> Switch4/2
  Switch4/1 -> Integrator/1
  Constant1/1 -> Switch3/1

== system RLFactory/RLServiceOpponentB/RLServiceAOpponentController/RLServiceEMAdjustVelocity ==
  MoveX : Inport
  MoveY : Inport  Port=2
  Velocity : Inport  Port=3
  Constant : Constant
  Demux1 : Demux  Outputs=2
  Divide : Product  Inputs=*/
  Divide1 : Product  Inputs=*/
  Mux : Mux  Inputs=2
  Product : Product
  Product3 : Product
  Sqrt1 : Sqrt  SaturateOnIntegerOverflow=on
  Square : Math  Operator=square  SaturateOnIntegerOverflow=on
  Square1 : Math  Operator=square  SaturateOnIntegerOverflow=on
  Sum : Sum  Inputs=+|+
  Switch : Switch  Criteria=u2 > Threshold
  AdjX : Outport
  AdjY : Outport  Port=2
  wires:
  Product/1 -> AdjX/1
  MoveY/1 -> Square1/1, Mux/2
  Mux/1 -> Demux1/1
  Divide1/1 -> Product3/1
  Constant/1 -> Switch/3
  Square1/1 -> Sum/2
  Switch/1 -> Divide1/2, Divide/2
  Velocity/1 -> Product/2, Product3/2
  Sum/1 -> Sqrt1/1
  Square/1 -> Sum/1
  Sqrt1/1 -> Switch/2, Switch/1
  Product3/1 -> AdjY/1
  Demux1/2 -> Divide1/1
  MoveX/1 -> Square/1, Mux/1
  Demux1/1 -> Divide/1
  Divide/1 -> Product/1

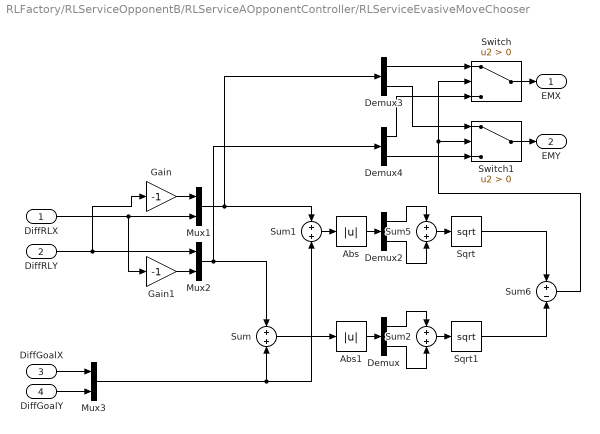
== system RLFactory/RLServiceOpponentB/RLServiceAOpponentController/RLServiceEvasiveMoveChooser ==
  DiffRLX : Inport
  DiffRLY : Inport  Port=2
  DiffGoalX : Inport  Port=3
  DiffGoalY : Inport  Port=4
  Abs : Abs
  Abs1 : Abs
  Demux{,2..4} (4 alike) : Demux  Outputs=2
  Gain : Gain  Gain=-1
  Gain1 : Gain  Gain=-1
  Mux1 : Mux  Inputs=2
  Mux2 : Mux  Inputs=2
  Mux3 : Mux  Inputs=2
  Sqrt : Sqrt  SaturateOnIntegerOverflow=on
  Sqrt1 : Sqrt  SaturateOnIntegerOverflow=on
  Sum{,1..2,5} (4 alike) : Sum  Inputs=+|+
  Sum6 : Sum  Inputs=+|-
  Switch : Switch  Criteria=u2 > Threshold
  Switch1 : Switch  Criteria=u2 > Threshold
  EMX : Outport
  EMY : Outport  Port=2
  wires:
  Gain/1 -> Mux1/1
  DiffRLX/1 -> Gain1/1, Mux1/2
  Gain1/1 -> Mux2/2
  DiffGoalX/1 -> Mux3/1
  DiffGoalY/1 -> Mux3/2
  Mux3/1 -> Sum/2, Sum1/2
  Mux2/1 -> Sum/1, Demux4/1
  Mux1/1 -> Demux3/1, Sum1/1
  Sum1/1 -> Abs/1
  Sum/1 -> Abs1/1
  Abs1/1 -> Demux/1
  Demux/1 -> Sum2/1
  Demux/2 -> Sum2/2
  Demux2/2 -> Sum5/2
  Demux2/1 -> Sum5/1
  Abs/1 -> Demux2/1
  Sum5/1 -> Sqrt/1
  Sum2/1 -> Sqrt1/1
  Sqrt/1 -> Sum6/1
  Sqrt1/1 -> Sum6/2
  Sum6/1 -> Switch/2, Switch1/2
  Demux3/1 -> Switch/1
  Demux3/2 -> Switch1/1
  Demux4/1 -> Switch/3
  Demux4/2 -> Switch1/3
  Switch/1 -> EMX/1
  Switch1/1 -> EMY/1
  DiffRLY/1 -> Mux2/1, Gain/1

== system RLFactory/RLServiceOpponentB/RLServiceAOpponentController/RLServiceInvalidMoveChecker ==
  MoveX : Inport
  MoveY : Inport  Port=2
  DiffRLX : Inport  Port=3
  DiffRLY : Inport  Port=4
  THRESHOLD : Inport  Port=5
  Constant5 : Constant
  Constant6 : Constant  Value=0
  Constant7 : Constant  Value=0
  Constant8 : Constant
  Constant9 : Constant
  Product : Product
  Product1 : Product
  Square : Math  Operator=square  SaturateOnIntegerOverflow=on
  Square Root : Sqrt  SaturateOnIntegerOverflow=on
  Square1 : Math  Operator=square  SaturateOnIntegerOverflow=on
  Sum : Sum  Inputs=+|-
  Sum1 : Sum
  Sum5 : Sum  Inputs=+|+
  Sum6 : Sum  Inputs=+|-|+
  Switch1 : Switch  Criteria=u2 > Threshold
  Switch3 : Switch  Criteria=u2 > Threshold
  MoveInValid : Outport
  wires:
  Product1/1 -> Sum5/2
  Sum5/1 -> Switch3/2
  Product/1 -> Sum5/1
  Sum6/1 -> MoveInValid/1
  Switch3/1 -> Sum6/1
  Constant9/1 -> Switch3/1
  MoveY/1 -> Product1/1
  MoveX/1 -> Product/1
  Constant8/1 -> Sum6/2
  Constant7/1 -> Switch3/3
  THRESHOLD/1 -> Sum/2
  Sum/1 -> Switch1/2
  Constant5/1 -> Switch1/3
  Constant6/1 -> Switch1/1
  Switch1/1 -> Sum6/3
  DiffRLY/1 -> Square1/1, Product1/2
  DiffRLX/1 -> Product/2, Square/1
  Square1/1 -> Sum1/2
  Sum1/1 -> Square Root/1
  Square/1 -> Sum1/1
  Square Root/1 -> Sum/1

== system RLFactory/RLServiceOpponentB/RLServiceAOpponentController/RLServicePMAdjustVelocity ==
  MoveX : Inport
  MoveY : Inport  Port=2
  Velocity : Inport  Port=3
  Constant : Constant
  Demux1 : Demux  Outputs=2
  Divide : Product  Inputs=*/
  Divide1 : Product  Inputs=*/
  Mux : Mux  Inputs=2
  Product : Product
  Product3 : Product
  Sqrt1 : Sqrt  SaturateOnIntegerOverflow=on
  Square : Math  Operator=square  SaturateOnIntegerOverflow=on
  Square1 : Math  Operator=square  SaturateOnIntegerOverflow=on
  Sum : Sum  Inputs=+|+
  Switch : Switch  Criteria=u2 > Threshold
  AdjX : Outport
  AdjY : Outport  Port=2
  wires:
  Velocity/1 -> Product/2, Product3/2
  MoveX/1 -> Square/1, Mux/1
  MoveY/1 -> Square1/1, Mux/2
  Divide1/1 -> Product3/1
  Divide/1 -> Product/1
  Switch/1 -> Divide1/2, Divide/2
  Constant/1 -> Switch/3
  Mux/1 -> Demux1/1
  Demux1/2 -> Divide1/1
  Square1/1 -> Sum/2
  Sum/1 -> Sqrt1/1
  Demux1/1 -> Divide/1
  Product/1 -> AdjX/1
  Sqrt1/1 -> Switch/2, Switch/1
  Product3/1 -> AdjY/1
  Square/1 -> Sum/1

== system RLFactory/RLServiceOpponentB/RLServiceAOpponentController/RLServiceXAvoidOvershooting ==
  MoveX : Inport
  MoveY : Inport  Port=2
  DiffToGoalX : Inport  Port=3
  DiffToGoalY : Inport  Port=4
  TS : Inport  Port=5
  Abs{1..4} (4 alike) : Abs
  Divide : Product  Inputs=*/
  Divide1 : Product  Inputs=*/
  Product : Product
  Product1 : Product
  Sum1 : Sum  Inputs=-|+
  Sum2 : Sum  Inputs=-|+
  Switch : Switch  Criteria=u2 > Threshold
  Switch1 : Switch  Criteria=u2 > Threshold
  MoveXNoOvershoot : Outport
  MoveYNoOvershoot : Outport  Port=2
  wires:
  Abs1/1 -> Sum1/2
  Switch/1 -> MoveXNoOvershoot/1
  Product/1 -> Abs2/1
  Abs2/1 -> Sum1/1
  DiffToGoalX/1 -> Divide/1, Abs1/1
  Sum1/1 -> Switch/2
  MoveX/1 -> Product/1, Switch/1
  Divide/1 -> Switch/3
  MoveY/1 -> Product1/1, Switch1/1
  Sum2/1 -> Switch1/2
  Abs4/1 -> Sum2/1
  Product1/1 -> Abs4/1
  Divide1/1 -> Switch1/3
  TS/1 -> Divide1/2, Product1/2, Divide/2, Product/2
  Abs3/1 -> Sum2/2
  Switch1/1 -> MoveYNoOvershoot/1
  DiffToGoalY/1 -> Divide1/1, Abs3/1

== system RLFactory/RLServiceRLRobot/RLServiceRLInfo/RLServiceCrashDetector ==
  X : Inport
  Y : Inport  Port=2
  AX : Inport  Port=3
  AY : Inport  Port=4
  BX : Inport  Port=5
  BY : Inport  Port=6
  Constant : Constant  Value=SAFETYDISTANCEA
  Constant1 : Constant  Value=SAFETYDISTANCEB
  Constant2 : Constant  Value=THRESHOLDA
  Constant3 : Constant  Value=THRESHOLDB
  Less Than{1..4} (4 alike) : RelationalOperator  Operator=<=  OutDataTypeStr=boolean  RndMeth=Simplest
  Memory : Memory
  OR : Logic  Operator=OR  IconShape=distinctive  AllPortsSameDT=off  OutDataTypeStr=boolean
  OR1 : Logic  Operator=OR  IconShape=distinctive  AllPortsSameDT=off  OutDataTypeStr=boolean
  RLServiceEuclideanDistanceCalculator1 : Subsystem
  RLServiceEuclideanDistanceCalculator2 : Subsystem
  Switch3 : Switch  Criteria=u2 > Threshold
  BelowThreshold : Outport
  Crash : Outport  Port=2
  wires:
  AX/1 -> RLServiceEuclideanDistanceCalculator1/3(XOpp)
  Less Than2/1 -> OR/1
  Memory/1 -> Switch3/1, Switch3/2
  Constant/1 -> Less Than2/2
  Y/1 -> RLServiceEuclideanDistanceCalculator2/2(Y), RLServiceEuclideanDistanceCalculator1/2(Y)
  AY/1 -> RLServiceEuclideanDistanceCalculator1/4(YOpp)
  X/1 -> RLServiceEuclideanDistanceCalculator1/1(X), RLServiceEuclideanDistanceCalculator2/1(X)
  OR/1 -> Switch3/3
  Constant1/1 -> Less Than3/2
  BY/1 -> RLServiceEuclideanDistanceCalculator2/4(YOpp)
  Less Than3/1 -> OR/2
  BX/1 -> RLServiceEuclideanDistanceCalculator2/3(XOpp)
  Constant2/1 -> Less Than1/2
  RLServiceEuclideanDistanceCalculator1/1(Dist) -> Less Than2/1, Less Than1/1
  Constant3/1 -> Less Than4/2
  RLServiceEuclideanDistanceCalculator2/1(Dist) -> Less Than4/1, Less Than3/1
  Less Than1/1 -> OR1/1
  Less Than4/1 -> OR1/2
  Switch3/1 -> Crash/1, Memory/1
  OR1/1 -> BelowThreshold/1

== system RLFactory/RLServiceRLRobot/RLServiceRLInfo/RLServiceGoalTracker ==
  X : Inport
  Y : Inport  Port=2
  GoalX : Inport  Port=3
  GoalY : Inport  Port=4
  Constant1 : Constant
  Constant5 : Constant  Value=0.5
  Constant7 : Constant  Value=0
  Less Than1 : RelationalOperator  Operator=<  OutDataTypeStr=boolean  RndMeth=Simplest
  RLServiceEuclideanDistanceCalculator : Subsystem
  Sum : Sum  Inputs=|++
  Switch : Switch  Criteria=u2 > Threshold
  To Workspace : ToWorkspace  VariableName=Arrived  SampleTime=TSRL
      settings: MaxDataPoints=1
  Unit Delay : UnitDelay  SampleTime=TSRL  HasFrameUpgradeWarning=on
  Zero-Order Hold : ZeroOrderHold  SampleTime=TSRL
  Dist : Outport
  Arrived : Outport  Port=2
  wires:
  Constant7/1 -> Switch/3
  GoalX/1 -> RLServiceEuclideanDistanceCalculator/3(GoalX)
  Y/1 -> RLServiceEuclideanDistanceCalculator/2(Y)
  RLServiceEuclideanDistanceCalculator/1(DistGoal) -> Dist/1, Less Than1/1
  Constant1/1 -> Switch/1
  Switch/1 -> Zero-Order Hold/1
  Less Than1/1 -> Switch/2
  X/1 -> RLServiceEuclideanDistanceCalculator/1(X)
  GoalY/1 -> RLServiceEuclideanDistanceCalculator/4(GoalY)
  Constant5/1 -> Less Than1/2
  Zero-Order Hold/1 -> Sum/1, Arrived/1
  Sum/1 -> Unit Delay/1, To Workspace/1
  Unit Delay/1 -> Sum/2

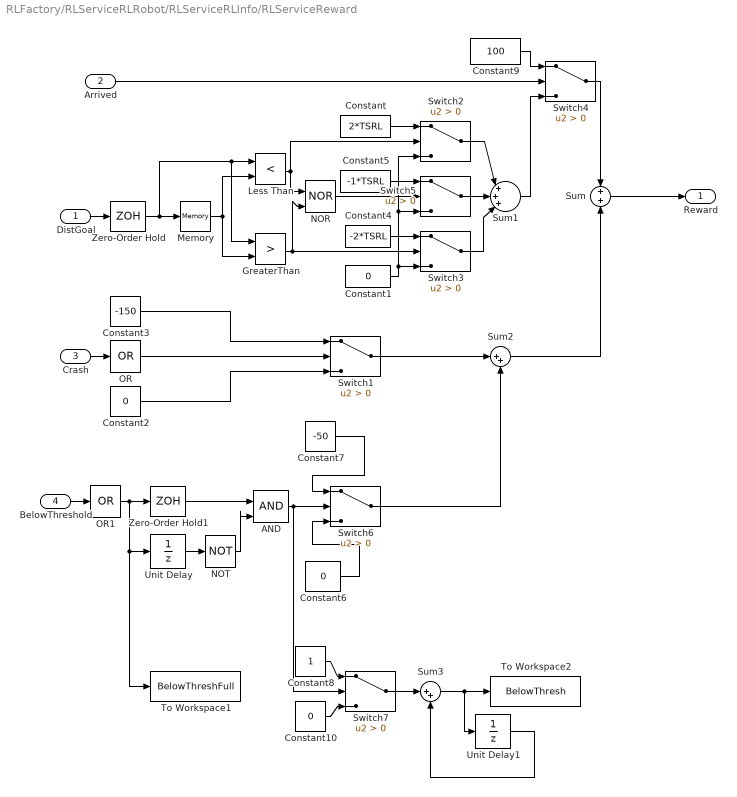
== system RLFactory/RLServiceRLRobot/RLServiceRLInfo/RLServiceReward ==
  DistGoal : Inport
  Arrived : Inport  Port=2
  Crash : Inport  Port=3
  BelowThreshold : Inport  Port=4
  AND : Logic  IconShape=distinctive  AllPortsSameDT=off  OutDataTypeStr=boolean
  Constant : Constant  Value=2*TSRL
  Constant{1..2,6,10} (4 alike) : Constant  Value=0
  Constant3 : Constant  Value=-150  VectorParams1D=off
  Constant4 : Constant  Value=-2*TSRL
  Constant5 : Constant  Value=-1*TSRL
  Constant7 : Constant  Value=-50  VectorParams1D=off
  Constant8 : Constant
  Constant9 : Constant  Value=100
  GreaterThan : RelationalOperator  Operator=>  OutDataTypeStr=boolean  RndMeth=Simplest
  Less Than : RelationalOperator  Operator=<  OutDataTypeStr=boolean  RndMeth=Simplest
  Memory : Memory
  NOR : Logic  Operator=NOR  IconShape=distinctive  AllPortsSameDT=off  OutDataTypeStr=boolean
  NOT : Logic  Operator=NOT  IconShape=distinctive  AllPortsSameDT=off  OutDataTypeStr=boolean
  OR : Logic  Operator=OR  Inputs=1  IconShape=distinctive  AllPortsSameDT=off  OutDataTypeStr=boolean
  OR1 : Logic  Operator=OR  Inputs=1  IconShape=distinctive  AllPortsSameDT=off  OutDataTypeStr=boolean
  Sum : Sum
  Sum1 : Sum  Inputs=|+++|
  Sum2 : Sum  Inputs=|++
  Sum3 : Sum  Inputs=|++
  Switch{1..7} (7 alike) : Switch  Criteria=u2 > Threshold
  To Workspace1 : ToWorkspace  VariableName=BelowThreshFull  SampleTime=TSRL
  To Workspace2 : ToWorkspace  VariableName=BelowThresh  SampleTime=TSRL
      settings: MaxDataPoints=1
  Unit Delay : UnitDelay  SampleTime=TSRL  HasFrameUpgradeWarning=on
  Unit Delay1 : UnitDelay  SampleTime=TSRL  HasFrameUpgradeWarning=on
  Zero-Order Hold : ZeroOrderHold  SampleTime=TSRL
  Zero-Order Hold1 : ZeroOrderHold  SampleTime=TSRL
  Reward : Outport
  wires:
  Sum/1 -> Reward/1
  Constant2/1 -> Switch1/3
  Constant3/1 -> Switch1/1
  Sum2/1 -> Sum/2
  DistGoal/1 -> Zero-Order Hold/1
  Memory/1 -> GreaterThan/2, Less Than/2
  Switch4/1 -> Sum/1
  Constant9/1 -> Switch4/1
  Switch2/1 -> Sum1/1
  Arrived/1 -> Switch4/2
  OR/1 -> Switch1/2
  Less Than/1 -> NOR/1, Switch2/2
  Constant/1 -> Switch2/1
  Constant1/1 -> Switch2/3, Switch5/3, Switch3/3
  GreaterThan/1 -> NOR/2, Switch3/2
  Constant4/1 -> Switch3/1
  Sum1/1 -> Switch4/3
  Switch3/1 -> Sum1/3
  NOR/1 -> Switch5/2
  Constant5/1 -> Switch5/1
  Switch5/1 -> Sum1/2
  Zero-Order Hold/1 -> Memory/1, GreaterThan/1, Less Than/1
  Crash/1 -> OR/1
  OR1/1 -> Zero-Order Hold1/1, To Workspace1/1, Unit Delay/1
  Constant7/1 -> Switch6/1
  BelowThreshold/1 -> OR1/1
  Constant6/1 -> Switch6/3
  Switch6/1 -> Sum2/2
  Switch1/1 -> Sum2/1
  Unit Delay/1 -> NOT/1
  NOT/1 -> AND/2
  Sum3/1 -> To Workspace2/1, Unit Delay1/1
  Zero-Order Hold1/1 -> AND/1
  Unit Delay1/1 -> Sum3/2
  Switch7/1 -> Sum3/1
  Constant8/1 -> Switch7/1
  Constant10/1 -> Switch7/3
  AND/1 -> Switch7/2, Switch6/2

== system RLFactory/RLServiceRLRobot/RLServiceRLMotorControl/RLServiceRLAdjustVelocity ==
  MoveX : Inport
  MoveY : Inport  Port=2
  Velocity : Inport  Port=3
  Constant : Constant
  Demux1 : Demux  Outputs=2
  Divide : Product  Inputs=*/
  Divide1 : Product  Inputs=*/
  Mux : Mux  Inputs=2
  Product : Product
  Product3 : Product
  Sqrt1 : Sqrt  SaturateOnIntegerOverflow=on
  Square : Math  Operator=square  SaturateOnIntegerOverflow=on
  Square1 : Math  Operator=square  SaturateOnIntegerOverflow=on
  Sum : Sum  Inputs=+|+
  Switch : Switch  Criteria=u2 > Threshold
  AdjMX : Outport
  AdjMY : Outport  Port=2
  wires:
  Product/1 -> AdjMX/1
  MoveY/1 -> Square1/1, Mux/2
  Mux/1 -> Demux1/1
  Divide1/1 -> Product3/1
  Constant/1 -> Switch/3
  Square1/1 -> Sum/2
  Switch/1 -> Divide1/2, Divide/2
  Velocity/1 -> Product/2, Product3/2
  Sum/1 -> Sqrt1/1
  Square/1 -> Sum/1
  Sqrt1/1 -> Switch/2, Switch/1
  Product3/1 -> AdjMY/1
  Demux1/2 -> Divide1/1
  MoveX/1 -> Square/1, Mux/1
  Demux1/1 -> Divide/1
  Divide/1 -> Product/1

== system RLFactory/RLServiceRLRobot/RLServiceRLRobotSensor/RLServiceARobotSensorSubsystem ==
  X : Inport
  Y : Inport  Port=2
  OppX : Inport  Port=3
  OppY : Inport  Port=4
  Demux4 : Demux  Outputs=2
  Demux6 : Demux  Outputs=2
  Mux : Mux  Inputs=2
  Mux1 : Mux  Inputs=2
  RLServiceDirectionCalculator : Subsystem
  Sum : Sum  Inputs=-+|
  DiffOppX : Outport
  DiffOppY : Outport  Port=2
  DirOppX : Outport  Port=3
  DirOppY : Outport  Port=4
  wires:
  Mux/1 -> Sum/2, Demux6/1
  Demux6/2 -> RLServiceDirectionCalculator/2(OppY)
  OppX/1 -> Mux/1
  X/1 -> Mux1/1
  Y/1 -> Mux1/2
  Demux6/1 -> RLServiceDirectionCalculator/1(OppX)
  RLServiceDirectionCalculator/1(DirOppX) -> DirOppX/1
  OppY/1 -> Mux/2
  Mux1/1 -> Sum/1
  Sum/1 -> Demux4/1
  RLServiceDirectionCalculator/2(DirOppY) -> DirOppY/1
  Demux4/1 -> DiffOppX/1
  Demux4/2 -> DiffOppY/1

== system RLFactory/RLServiceRLRobot/RLServiceRLRobotSensor/RLServiceBRobotSensorSubsystem ==
  X : Inport
  Y : Inport  Port=2
  OppX : Inport  Port=3
  OppY : Inport  Port=4
  Demux4 : Demux  Outputs=2
  Demux6 : Demux  Outputs=2
  Mux : Mux  Inputs=2
  Mux1 : Mux  Inputs=2
  RLServiceDirectionCalculator : Subsystem
  Sum : Sum  Inputs=-+|
  DiffOppX : Outport
  DiffOppY : Outport  Port=2
  DirOppX : Outport  Port=3
  DirOppY : Outport  Port=4
  wires:
  Mux/1 -> Sum/2, Demux6/1
  Demux6/2 -> RLServiceDirectionCalculator/2(OppY)
  OppX/1 -> Mux/1
  X/1 -> Mux1/1
  Y/1 -> Mux1/2
  Demux6/1 -> RLServiceDirectionCalculator/1(OppX)
  RLServiceDirectionCalculator/1(DirOppX) -> DirOppX/1
  OppY/1 -> Mux/2
  Mux1/1 -> Sum/1
  Sum/1 -> Demux4/1
  RLServiceDirectionCalculator/2(DirOppY) -> DirOppY/1
  Demux4/1 -> DiffOppX/1
  Demux4/2 -> DiffOppY/1

== system RLFactory/RLServiceOpponentA/RLServiceAOpponentController/RLServiceArrivedChecker/RLServiceEuclideanDistanceCalculator1 ==
  X : Inport
  Y : Inport  Port=2
  GoalX : Inport  Port=3
  GoalY : Inport  Port=4
  Square : Math  Operator=square  SaturateOnIntegerOverflow=on
  Square Root : Sqrt  SaturateOnIntegerOverflow=on
  Square1 : Math  Operator=square  SaturateOnIntegerOverflow=on
  Sum1 : Sum
  Sum3 : Sum  Inputs=+-
  Sum4 : Sum  Inputs=+-
  DistToGoal : Outport
  wires:
  GoalX/1 -> Sum3/2
  X/1 -> Sum3/1
  Sum1/1 -> Square Root/1
  Sum4/1 -> Square1/1
  Square/1 -> Sum1/1
  Y/1 -> Sum4/1
  Square Root/1 -> DistToGoal/1
  Square1/1 -> Sum1/2
  Sum3/1 -> Square/1
  GoalY/1 -> Sum4/2

== system RLFactory/RLServiceOpponentA/RLServiceAOpponentController/RLServiceArrivedChecker/RLServiceEuclideanDistanceCalculator2 ==
  X : Inport
  Y : Inport  Port=2
  GoalX : Inport  Port=3
  GoalY : Inport  Port=4
  Square : Math  Operator=square  SaturateOnIntegerOverflow=on
  Square Root : Sqrt  SaturateOnIntegerOverflow=on
  Square1 : Math  Operator=square  SaturateOnIntegerOverflow=on
  Sum1 : Sum
  Sum3 : Sum  Inputs=+-
  Sum4 : Sum  Inputs=+-
  OppDistToGoal : Outport
  wires:
  GoalX/1 -> Sum3/2
  X/1 -> Sum3/1
  Sum1/1 -> Square Root/1
  Sum4/1 -> Square1/1
  Square/1 -> Sum1/1
  Y/1 -> Sum4/1
  Square Root/1 -> OppDistToGoal/1
  Square1/1 -> Sum1/2
  Sum3/1 -> Square/1
  GoalY/1 -> Sum4/2

== system RLFactory/RLServiceOpponentB/RLServiceAOpponentController/RLServiceArrivedChecker/RLServiceEuclideanDistanceCalculator1 ==
  X : Inport
  Y : Inport  Port=2
  GoalX : Inport  Port=3
  GoalY : Inport  Port=4
  Square : Math  Operator=square  SaturateOnIntegerOverflow=on
  Square Root : Sqrt  SaturateOnIntegerOverflow=on
  Square1 : Math  Operator=square  SaturateOnIntegerOverflow=on
  Sum1 : Sum
  Sum3 : Sum  Inputs=+-
  Sum4 : Sum  Inputs=+-
  DistToGoal : Outport
  wires:
  GoalX/1 -> Sum3/2
  X/1 -> Sum3/1
  Sum1/1 -> Square Root/1
  Sum4/1 -> Square1/1
  Square/1 -> Sum1/1
  Y/1 -> Sum4/1
  Square Root/1 -> DistToGoal/1
  Square1/1 -> Sum1/2
  Sum3/1 -> Square/1
  GoalY/1 -> Sum4/2

== system RLFactory/RLServiceOpponentB/RLServiceAOpponentController/RLServiceArrivedChecker/RLServiceEuclideanDistanceCalculator2 ==
  X : Inport
  Y : Inport  Port=2
  GoalX : Inport  Port=3
  GoalY : Inport  Port=4
  Square : Math  Operator=square  SaturateOnIntegerOverflow=on
  Square Root : Sqrt  SaturateOnIntegerOverflow=on
  Square1 : Math  Operator=square  SaturateOnIntegerOverflow=on
  Sum1 : Sum
  Sum3 : Sum  Inputs=+-
  Sum4 : Sum  Inputs=+-
  OppDistToGoal : Outport
  wires:
  GoalX/1 -> Sum3/2
  X/1 -> Sum3/1
  Sum1/1 -> Square Root/1
  Sum4/1 -> Square1/1
  Square/1 -> Sum1/1
  Y/1 -> Sum4/1
  Square Root/1 -> OppDistToGoal/1
  Square1/1 -> Sum1/2
  Sum3/1 -> Square/1
  GoalY/1 -> Sum4/2

== system RLFactory/RLServiceRLRobot/RLServiceRLInfo/RLServiceCrashDetector/RLServiceEuclideanDistanceCalculator1 ==
  X : Inport
  Y : Inport  Port=2
  XOpp : Inport  Port=3
  YOpp : Inport  Port=4
  Square : Math  Operator=square  SaturateOnIntegerOverflow=on
  Square Root : Sqrt  SaturateOnIntegerOverflow=on
  Square1 : Math  Operator=square  SaturateOnIntegerOverflow=on
  Sum1 : Sum
  Sum3 : Sum  Inputs=+-
  Sum4 : Sum  Inputs=+-
  Dist : Outport
  wires:
  XOpp/1 -> Sum3/2
  X/1 -> Sum3/1
  Sum1/1 -> Square Root/1
  Sum4/1 -> Square1/1
  Square/1 -> Sum1/1
  Y/1 -> Sum4/1
  Square Root/1 -> Dist/1
  Square1/1 -> Sum1/2
  Sum3/1 -> Square/1
  YOpp/1 -> Sum4/2
